simulink model "SwarmSystem"  (R2022b)
settings: Solver=VariableStepAuto  StartTime=0.0  StopTime=10.0  RelTol=1e-3
values from neighbouring files (symbols this model uses):
  dt = 0.01    [init_params.m]
  initial_state_x0 = Simulink.Parameter(initial_state_x0)    [init_params.m]    (also in single_model_verification_script.m = [W0; R0; dP0; P0]; team_model_conf_comp_script.m = [W0; R0; dP0; P0]; team_model_tethered_tilt.m = [W0; R0; dP0; P0]; team_model_tracking_script.m = [W0; R0; dP0; P0])
undefined symbols (not defined in the file or in its folder): drone_params, env_params
libraries: dspindex x15, aerolibanim x1
(part 1 of 4)
settings Model: Creator=NTU  LastModifiedBy=NTU

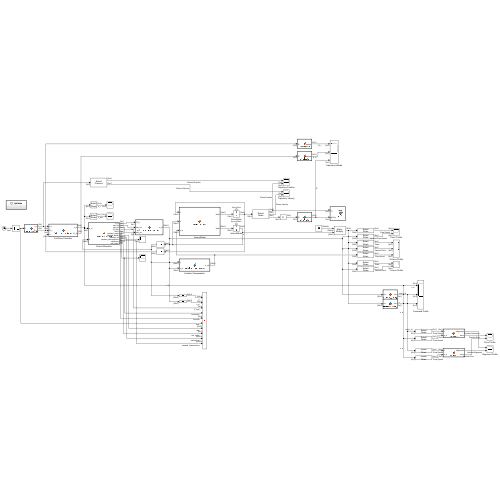
[thumbnail: Simulink's stored preview of the top-level diagram]
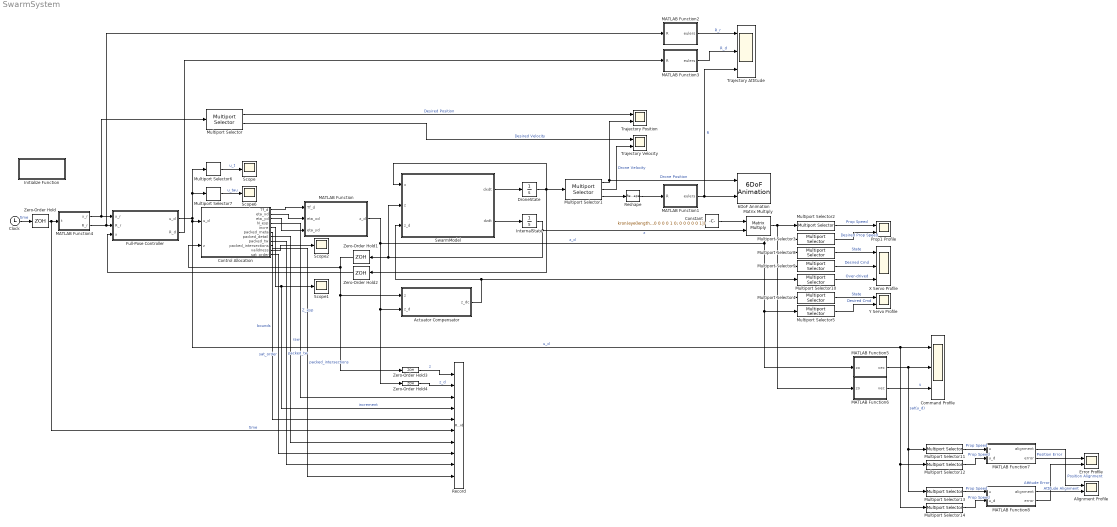
== system SwarmSystem ==
  6DoF Animation : aerolibanim/6DoF Animation  u1=[-10 10 0 20 -10 10]  u2=0.1  u3=1.0  u4=[0 10 0]  u5=Fixed position  u6=[20 20 20]  u7=-40  u8=on
  Actuator Compensator : MATLAB Function  TreatAsAtomicUnit=on
  Alignment Profile : Scope  NumInputPorts=2
  Clock : Clock
  Command Profile : Scope  NumInputPorts=3
  Constant : Constant  Value=kron(eye(length(drone_params.psi)), [1 0 0 0 0 0;0 0 1 0 0 0; 0 0 0 0 1 0; 0 0 0 0 0 1])  VectorParams1D=off
  Control Allocation : MATLAB Function  TreatAsAtomicUnit=on
  DroneState : Integrator  InitialCondition=zeros([18 1])
  Error Profile : Scope  NumInputPorts=2
  Full-Pose Controller : MATLAB Function  TreatAsAtomicUnit=on
  Initialize Function : Subsystem  TreatAsAtomicUnit=on
  InternalState : Integrator  InitialCondition=zeros([6*length(drone_params.psi) 1])
  MATLAB Function : MATLAB Function  TreatAsAtomicUnit=on
  MATLAB Function1 : MATLAB Function  TreatAsAtomicUnit=on
  MATLAB Function2 : MATLAB Function  TreatAsAtomicUnit=on
  MATLAB Function3 : MATLAB Function  TreatAsAtomicUnit=on
  MATLAB Function4 : MATLAB Function  TreatAsAtomicUnit=on
  MATLAB Function5 : MATLAB Function  TreatAsAtomicUnit=on
  MATLAB Function6 : MATLAB Function  TreatAsAtomicUnit=on
  MATLAB Function7 : MATLAB Function  TreatAsAtomicUnit=on
  MATLAB Function8 : MATLAB Function  TreatAsAtomicUnit=on
  Matrix Multiply : Product  Multiplication=Matrix(*)
  Multiport Selector : dspindex/Multiport Selector  rowsOrCols=Columns  idxCellArray={ 1, 2 }  idxErrMode=Clip Index
  Multiport Selector1 : dspindex/Multiport Selector  rowsOrCols=Rows  idxCellArray={ [16:18], [13:15], [4:12] }  idxErrMode=Clip Index
  Multiport Selector10 : dspindex/Multiport Selector  rowsOrCols=Rows  idxCellArray={ [4 8 12 16 20 24 28 32 36]-3 }  idxErrMode=Clip Index
  Multiport Selector11 : dspindex/Multiport Selector  rowsOrCols=Rows  idxCellArray={ [1:3]}  idxErrMode=Clip Index
  Multiport Selector12 : dspindex/Multiport Selector  rowsOrCols=Rows  idxCellArray={ [1:3]}  idxErrMode=Clip Index
  Multiport Selector13 : dspindex/Multiport Selector  rowsOrCols=Rows  idxCellArray={ [4:6]}  idxErrMode=Clip Index
  Multiport Selector14 : dspindex/Multiport Selector  rowsOrCols=Rows  idxCellArray={ [4:6]}  idxErrMode=Clip Index
  Multiport Selector2 : dspindex/Multiport Selector  rowsOrCols=Rows  idxCellArray={ [4 8 12 16 20 24 28 32 36]-1 }  idxErrMode=Clip Index
  Multiport Selector3 : dspindex/Multiport Selector  rowsOrCols=Rows  idxCellArray={ [4 8 12 16 20 24 28 32 36]-1 }  idxErrMode=Clip Index
  Multiport Selector4 : dspindex/Multiport Selector  rowsOrCols=Rows  idxCellArray={ [4 8 12 16 20 24 28 32 36]-2 }  idxErrMode=Clip Index
  Multiport Selector5 : dspindex/Multiport Selector  rowsOrCols=Rows  idxCellArray={ [4 8 12 16 20 24 28 32 36]-2 }  idxErrMode=Clip Index
  Multiport Selector6 : dspindex/Multiport Selector  rowsOrCols=Rows  idxCellArray={ [1:3] }  idxErrMode=Clip Index
  Multiport Selector7 : dspindex/Multiport Selector  rowsOrCols=Rows  idxCellArray={ [4:6] }  idxErrMode=Clip Index
  Multiport Selector8 : dspindex/Multiport Selector  rowsOrCols=Rows  idxCellArray={ [4 8 12 16 20 24 28 32 36]-3 }  idxErrMode=Clip Index
  Multiport Selector9 : dspindex/Multiport Selector  rowsOrCols=Rows  idxCellArray={ [4 8 12 16 20 24 28 32 36]-3 }  idxErrMode=Clip Index
  Prop1 Profile : Scope  NumInputPorts=2
